simulink model "CM680A_HwTq2Meas"  (R2013b)
settings: Solver=FixedStepDiscrete  SolverMode=SingleTasking  StartTime=0.0  StopTime=1  FixedStep=0.002  RelTol=1e-3
values from neighbouring files (symbols this model uses):
  ELECGLBPRM_HWTQOFFS_HWNWTMTR_F32 = DataDict.Constant    [CM680A_HwTq2Meas_DataDict.m]
  ELECGLBPRM_HWTQSATNLOWRLIM_HWNWTMTR_F32 = DataDict.Constant    [CM680A_HwTq2Meas_DataDict.m]
  ELECGLBPRM_HWTQSATNUPPRLIM_HWNWTMTR_F32 = DataDict.Constant    [CM680A_HwTq2Meas_DataDict.m]
  ELECGLBPRM_HWTQSCA_ULS_F32 = DataDict.Constant    [CM680A_HwTq2Meas_DataDict.m]
  ELECGLBPRM_NOFLT_CNT_U08 = DataDict.Constant    [CM680A_HwTq2Meas_DataDict.m]
  ELECGLBPRM_OFFSTRIMNOTPRFM_CNT_U08 = DataDict.Constant    [CM680A_HwTq2Meas_DataDict.m]
  ELECGLBPRM_PRTCLFLT_CNT_U08 = DataDict.Constant    [CM680A_HwTq2Meas_DataDict.m]
  ELECGLBPRM_SNSRINTFLT_CNT_U08 = DataDict.Constant    [CM680A_HwTq2Meas_DataDict.m]
  FLTINJ_HWTQ2MEAS_HWTQ2 = DataDict.Constant    [CM680A_HwTq2Meas_DataDict.m]
  GearIdn1 = DataDict.OpSignal    [CM680A_HwTq2Meas_DataDict.m]
  HwTq2MeasHwTq2PrtclFltFailStep = DataDict.Calibration    [CM680A_HwTq2Meas_DataDict.m]
  HwTq2MeasHwTq2PrtclFltPassStep = DataDict.Calibration    [CM680A_HwTq2Meas_DataDict.m]
undefined symbols (not defined in the file or in its folder): NtcNr1, NtcSts1, sigbuilder_block, SigQlfr1
libraries: simulink x22, NxtrNvM x3
(part 1 of 3)
settings Model: RequirementInfo={'doors' '00006115' '1' 'false' 'DOORS Surrogate Item' '' } %GIDa_184d7b6b_0c7e_41d3_b9a0_1a88eb3981d4  reqMgrSettings="100 S'doors','misc'{{S'surrogatepath','savemodel','savesurrogate','updateLinks','doorsLinks2sl','slLinks2Doors','purgeDoors','purgeSimulink','detaillevel','surrogateId','synctime'{{T\"/ESG Group/CM660A_HwTq1Meas\",M[1],M[1],M[0],M[0],M[1],M[0],M[0],M[1],T\"00006115\",T\"\"}},S'mode','pathStorage'{{T\"generic\",T\"modelRelative\"}}}}"  CovMetricSettings=dcmriw  CovFilter=CM680A_HwTq2Meas_covfilter  CovHTMLOptions=-sRT=0 -aTS=1 -bRG=1 -bTC=1 -hTR=0 -nFC=0 -scm=1 -bcm=1 -xEv=0  CovHtmlReporting=off  CovModelRefEnable=off  Creator=CZ68DS  LastModifiedBy=CZ68DS
settings SolverCC: AutoInsertRateTranBlk=on  InsertRTBMode=Always
settings DataIOCC: LimitDataPoints=off  SaveFormat=Structure  ReturnWorkspaceOutputs=on
settings OptimizationCC: BlockReduction=off  InlineParams=on  ZeroExternalMemoryAtStartup=off  ZeroInternalMemoryAtStartup=off  OptimizeModelRefInitCode=on  LifeSpan=1
settings DebuggingCC: SignalInfNanChecking=error  SignalRangeChecking=warning  UnderspecifiedInitializationDetection=Simplified  SolverPrmCheckMsg=error  InheritedTsInSrcMsg=error  DiscreteInheritContinuousMsg=error  SingleTaskRateTransMsg=error  TasksWithSamePriorityMsg=error  SigSpecEnsureSampleTimeMsg=error  CheckMatrixSingularityMsg=error  ParameterUnderflowMsg=error  ParameterPrecisionLossMsg=error  ParameterTunabilityLossMsg=error  FixptConstUnderflowMsg=warning  FixptConstOverflowMsg=warning  VectorMatrixConversionMsg=error  SignalLabelMismatchMsg=error  UnconnectedInputMsg=error  UnconnectedOutputMsg=error  UnconnectedLineMsg=error  SFcnCompatibilityMsg=error  UniqueDataStoreMsg=warning  BusObjectLabelMismatch=error  RootOutportRequireBusObject=error  AssertControl=DisableAll  ModelReferenceIOMsg=error  ModelReferenceVersionMismatchMessage=warning  ModelReferenceIOMismatchMessage=error  ModelReferenceCSMismatchMessage=warning  ModelReferenceDataLoggingMessage=error  StateNameClashWarn=warning  StrictBusMsg=ErrorOnBusTreatedAsVector  NonBusSignalsTreatedAsBus=error  SFUnexpectedBacktrackingDiag=error  SFInvalidInputDataAccessInChartInitDiag=error  SFNoUnconditionalDefaultTransitionDiag=error  SFTransitionOutsideNaturalParentDiag=error  SFUnconditionalTransitionShadowingDiag=error  SFUndirectedBroadcastEventsDiag=error
settings ModelReferenceCC: ModelReferenceNumInstancesAllowed=Single
settings RTWCC: SystemTargetFile=autosar.tlc  GenCodeOnly=on  TemplateMakefile=ert_default_tmf  Description=AUTOSAR  GenerateReport=on  ProcessScript=autosar_make_rtw_hook  LaunchReport=on
settings CodeAppCC: GenerateComments=off  IgnoreCustomStorageClasses=off  CustomSymbolStrType=$N$R$M  CustomSymbolStrBlkIO=$N$M  SimulinkBlockComments=off
settings STFCustomTargetCC: ParMdlRefBuildCompliant=on  CompOptLevelCompliant=on  IncludeMdlTerminateFcn=off  CombineOutputUpdateFcns=on  SuppressErrorStatus=on  ERTFirstTimeCompliant=on  ERTCustomFileBanners=on  SupportNonFinite=off  SupportComplex=off  SupportContinuousTime=off  SupportNonInlinedSFcns=off  MATLABClassNameForMDSCustomization=Simulink.SoftwareTarget.ERTCustomization  AutosarCompliant=on  GRTInterface=off  SystemTargetFile=autosar.tlc
settings ERTTargetCC: CodeReplacementLibrary=ANSI_C  ConcurrentExecutionCompliant=off  IncludeMdlTerminateFcn=off  SuppressErrorStatus=on  SupportNonFinite=off  SupportComplex=off  ModelStepFunctionPrototypeControlCompliant=off  CPPClassGenCompliant=off  AutosarCompliant=on  InlinedParameterPlacement=NonHierarchical  ERTCustomFileTemplate=example_file_process.tlc  EnableUserReplacementTypes=on

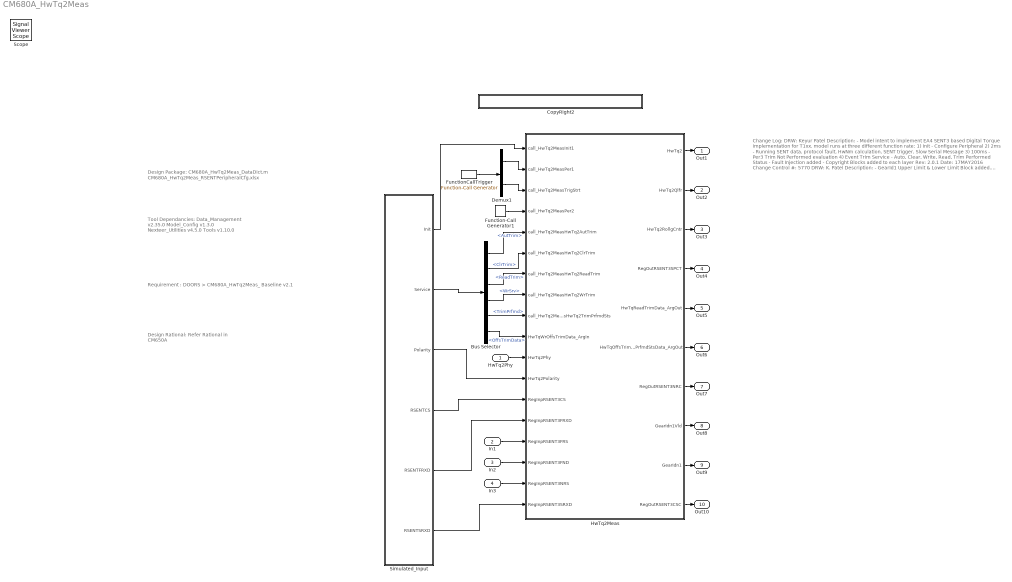
== system CM680A_HwTq2Meas ==
  note: Design Package:
      |
      | CM680A_HwTq2Meas_DataDict.m
      | CM680A_HwTq2Meas_RSENTPeripheralCfg.xlsx
  note: Change Log:
      |
      | DRW: Keyur Patel
      | Description:
      | - Model intent to implement EA4 SENT3 based Digital Torque implementation for T1xx.
      |    model runs at three different function rate:
      |       1) Init - Configure Peripheral
      |       2) 2ms - Running SENT data, protocol fault, HwNm calculation, SENT trigger, Slow Serial Message
      |       3) 100ms - Per3 Trim Not Performed evaluation
      |       4) Event Trim Service - Auto, Clear, Write, Read, Trim Performed Status
      | - Fault Injection added
      | - Copyright Blocks added to each layer
      |
      | Rev: 2.0.1
      | Date: 17MAY2016
      | Change Control #: 5770
      | DRW: K. Patel
      | Description:
      | - GearId1 Upper Limit & Lower Limit Block added.
      |
      | Rev: 2.0.0
      | Date: 15MAR2016
      | Change Control #: 4733
      | DRW: K. Patel
      | Description:
      | - Slow Serial Data Read Added for "C Factor & Bushing" signal read
      | - Timer 2us added before SPCT in NRS check added instead of SYNCM
      | - Refer Red Color High lighted Changes.
      |
      | Rev: 1.4.0
      | Date: 19JAN2016
      | Change Control #: 3376
      | DRW: K. Patel
      | Description:
      | - Refer Red Color High lighted Changes.
      | -  "CM680A_HwTq2Meas_RSENTPeripheralCfg.xlsx" change
      |
      | Rev: 1.3.0
      | Date: 16DEC2015
      | Change Control #: 3159
      | DRW: K. Patel
      | Description:
      | - Refer Red Color High lighted Changes.
      |
      | Rev: 1.2.0
      | Date: 09OCT2015
      | Change Control #: EA4#1923
      | DRW: K. Patel
      | Description:
      | - Torque Trigger server function, Per3 change to Per2, Missing Message Counter add per1,
      | remove register from "CM680A_HwTq2Meas_RSENTPeripheralCfg.xlsx", change sync time to 16
      |
      | Rev: 1.1.0
      | Date: 31JUL2015
      | Change Control #: WCR-EA4#1231
      | DRW: K. Patel
      | Description:
      | - m file correction, Tick Time change from 1us to 1.2us
      | - Global Constant
      |
      | Rev: 1.0.0
      | Date: 30JUN2015
      | Change Control #: WCR-EA4#1031
      | DRW: K. Patel
      | Description:
      | - Initial Release
      | - Fault Injection
      | - Trim Services Added
  note: Tool Dependancies:
      |
      | Data_Management v2.35.0
      | Model_Config v1.3.0
      | Nexteer_Utilities v4.5.0
      | Tools v1.10.0
  note: Requirement :
      |
      | DOORS > CM680A_HwTq2Meas_ Baseline v2.1
  note: Design Rational:
      |
      | Refer Rational in CM650A
  HwTq2Phy : Inport
  In1 : Inport  Port=2
  In2 : Inport  Port=3
  In3 : Inport  Port=4
  Bus Selector : BusSelector  OutputSignals=AutTrim,ClrTrim,ReadTrim,WrSrv,TrimPrfmd,OffsTrimData
  CopyRight2 : Subsystem  Description=|  mask(Copyright Information){none=on}
      | Copyright info block.                                               
      |                                                                     
      | Place copyright information at the top of every subsystem in design.
      mask prompts: none "No parameters"
      mask help: Place copyright information at the top of every subsystem in design.
      mask Display:
      | NxtrConf = 'Nexteer Confidential';
      | 
      | sys = bdroot; %handle for the current model ("system")
      | first = get_param(sys,'Created');
      | first = first(end-3:end);  %year is last four digits
      | 
      | last = get_param(sys,'LastModifiedDate');
      | if isempty(last)
      |     last = datestr(now,'yyyy');
      | else
      |     last = last(end-3:end);
      | end
      | 
      | if strcmp(first,last)
      |     fprintf('%s -- Copyright %s Nexteer',NxtrConf,first)
      | else
      |     fprintf('%s -- %s%s- %s Nexteer',NxtrConf,char(169),first,last)
      | end
  Demux1 : Demux  Outputs=2
  Function-Call Generator1 : simulink/Ports & Subsystems/Function-Call Generator  sample_time=0.100  numberOfIterations=1
  FunctionCallTrigger : simulink/Ports & Subsystems/Function-Call Generator  RequirementInfo={} %GIDa_461051ca_e299_4da2_91c0_e73e41056377  sample_time=0.002  numberOfIterations=1
  HwTq2Meas : Subsystem  RequirementInfo={'doors' '00006115' '2' 'false' 'DOORS Surrogate Item' '' } %GIDa_76d712c1_5f1a_450e_83af_7c4f481758f4  Priority=1
      settings: AttributesFormatString=Priority = %<Priority>
  Simulated_Input : Subsystem  Description=Do not Code this block
      settings: AttributesFormatString=%<Description>
  Out1 : Outport
  Out2 : Outport  Port=2
  Out3 : Outport  Port=3
  Out4 : Outport  Port=4
  Out5 : Outport  Port=5
  Out6 : Outport  Port=6
  Out7 : Outport  Port=7
  Out8 : Outport  Port=8
  Out9 : Outport  Port=9
  Out10 : Outport  Port=10
  Scope : SignalViewerScope  IOType=viewer  RefreshTime=0.035000
  wires:
  FunctionCallTrigger/1 -> Demux1/1
  HwTq2Phy/1 -> HwTq2Meas/11(HwTq2Phy)
  Simulated_Input/3(Polarity) -> HwTq2Meas/12(HwTq2Polarity)
  HwTq2Meas/3(HwTq2RollgCntr) -> Out3/1
  HwTq2Meas/1(HwTq2) -> Out1/1
  HwTq2Meas/2(HwTq2Qlfr) -> Out2/1
  HwTq2Meas/4(RegOutRSENT3SPCT) -> Out4/1
  Function-Call Generator1/1 -> HwTq2Meas/4(call_HwTq2MeasPer2)
  Demux1/1 -> HwTq2Meas/2(call_HwTq2MeasPer1)
  Demux1/2 -> HwTq2Meas/3(call_HwTq2MeasTrigStrt)
  Bus Selector/1 -> HwTq2Meas/5(call_HwTq2MeasHwTq2AutTrim)  "<AutTrim>"
  Bus Selector/2 -> HwTq2Meas/6(call_HwTq2MeasHwTq2ClrTrim)  "<ClrTrim>"
  Bus Selector/3 -> HwTq2Meas/7(call_HwTq2MeasHwTq2ReadTrim)  "<ReadTrim>"
  Bus Selector/4 -> HwTq2Meas/8(call_HwTq2MeasHwTq2WrTrim)  "<WrSrv>"
  Bus Selector/5 -> HwTq2Meas/9(call_HwTq2MeasHwTq2TrimPrfmdSts)  "<TrimPrfmd>"
  Bus Selector/6 -> HwTq2Meas/10(HwTqWrOffsTrimData_ArgIn)  "<OffsTrimData>"
  Simulated_Input/1(Init) -> HwTq2Meas/1(call_HwTq2MeasInit1)
  Simulated_Input/2(Service) -> Bus Selector/1
  Simulated_Input/4(RSENTCS) -> HwTq2Meas/13(RegInpRSENT3CS)
  Simulated_Input/5(RSENTFRXD) -> HwTq2Meas/14(RegInpRSENT3FRXD)
  HwTq2Meas/5(HwTqReadTrimData_ArgOut) -> Out5/1
  HwTq2Meas/6(HwTqOffsTrimPrfmdStsData_ArgOut) -> Out6/1
  HwTq2Meas/7(RegOutRSENT3NRC) -> Out7/1
  In1/1 -> HwTq2Meas/15(RegInpRSENT3FRS)
  In2/1 -> HwTq2Meas/16(RegInpRSENT3FND)
  In3/1 -> HwTq2Meas/17(RegInpRSENT3NRS)
  Simulated_Input/6(RSENTSRXD) -> HwTq2Meas/18(RegInpRSENT3SRXD)
  HwTq2Meas/8(GearIdn1Vld) -> Out8/1
  HwTq2Meas/9(GearIdn1) -> Out9/1
  HwTq2Meas/10(RegOutRSENT3CSC) -> Out10/1

== system CM680A_HwTq2Meas/CopyRight2 ==

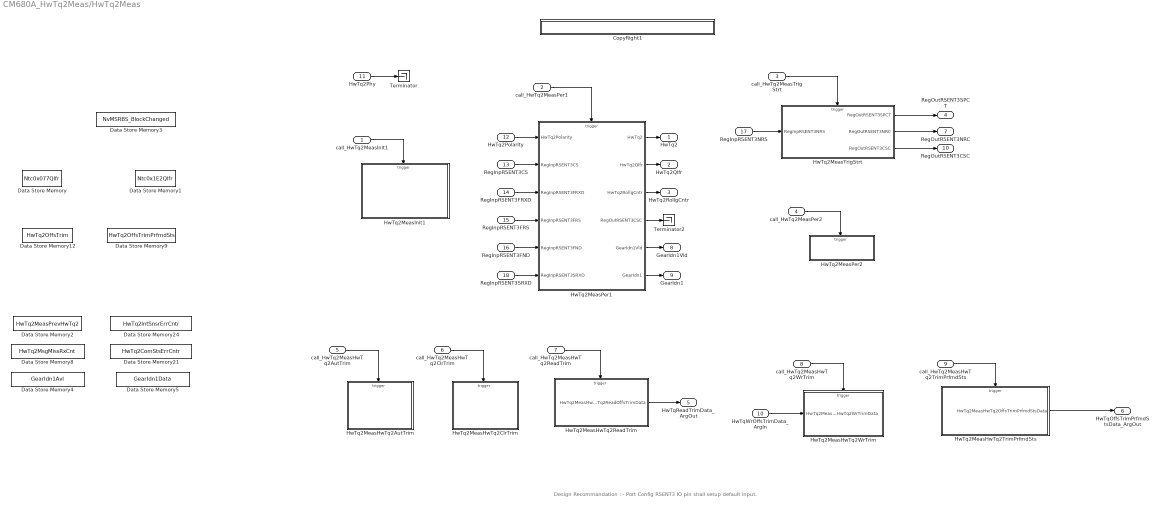
== system CM680A_HwTq2Meas/HwTq2Meas ==
  note: Design Recommandation :
      |
      | - Port Config RSENT3 IO pin shall setup default input.
  call_HwTq2MeasInit1 : Inport
  call_HwTq2MeasPer1 : Inport  Description=2ms  Port=2
      settings: AttributesFormatString=%<Description>
  call_HwTq2MeasTrigStrt : Inport  Description=Event  Port=3
      settings: AttributesFormatString=%<Description>
  call_HwTq2MeasPer2 : Inport  Description=100ms  Port=4
      settings: AttributesFormatString=%<Description>
  call_HwTq2MeasHwTq2AutTrim : Inport  Description=Event  Port=5
      settings: AttributesFormatString=%<Description>
  call_HwTq2MeasHwTq2ClrTrim : Inport  Description=Event  Port=6
      settings: AttributesFormatString=%<Description>
  call_HwTq2MeasHwTq2ReadTrim : Inport  Description=Event  Port=7
      settings: AttributesFormatString=%<Description>
  call_HwTq2MeasHwTq2WrTrim : Inport  Description=Event  Port=8
      settings: AttributesFormatString=%<Description>
  call_HwTq2MeasHwTq2TrimPrfmdSts : Inport  Description=Event  Port=9
      settings: AttributesFormatString=%<Description>
  HwTqWrOffsTrimData_ArgIn : Inport  Port=10
  HwTq2Phy : Inport  Port=11
  HwTq2Polarity : Inport  Port=12  OutDataTypeStr=int8
  RegInpRSENT3CS : Inport  Port=13
  RegInpRSENT3FRXD : Inport  Port=14
  RegInpRSENT3FRS : Inport  Port=15
  RegInpRSENT3FND : Inport  Port=16
  RegInpRSENT3NRS : Inport  Port=17
  RegInpRSENT3SRXD : Inport  Port=18
  CopyRight1 : Subsystem  Description=|  mask(Copyright Information){none=on}
      | Copyright info block.                                               
      |                                                                     
      | Place copyright information at the top of every subsystem in design.
      mask prompts: none "No parameters"
      mask help: Place copyright information at the top of every subsystem in design.
      mask Display:
      | NxtrConf = 'Nexteer Confidential';
      | 
      | sys = bdroot; %handle for the current model ("system")
      | first = get_param(sys,'Created');
      | first = first(end-3:end);  %year is last four digits
      | 
      | last = get_param(sys,'LastModifiedDate');
      | if isempty(last)
      |     last = datestr(now,'yyyy');
      | else
      |     last = last(end-3:end);
      | end
      | 
      | if strcmp(first,last)
      |     fprintf('%s -- Copyright %s Nexteer',NxtrConf,first)
      | else
      |     fprintf('%s -- %s%s- %s Nexteer',NxtrConf,char(169),first,last)
      | end
  Data Store Memory12 : DataStoreMemory  DataStoreName=HwTq2OffsTrim  ReadBeforeWriteMsg=warning  WriteAfterWriteMsg=warning  WriteAfterReadMsg=warning
  Data Store Memory2 : DataStoreMemory  DataStoreName=HwTq2MeasPrevHwTq2  ReadBeforeWriteMsg=warning  WriteAfterWriteMsg=warning  WriteAfterReadMsg=warning  StateMustResolveToSignalObject=on
  Data Store Memory21 : DataStoreMemory  DataStoreName=HwTq2ComStsErrCntr  ReadBeforeWriteMsg=warning  WriteAfterWriteMsg=warning  WriteAfterReadMsg=warning  StateMustResolveToSignalObject=on
  Data Store Memory24 : DataStoreMemory  DataStoreName=HwTq2IntSnsrErrCntr  ReadBeforeWriteMsg=warning  WriteAfterWriteMsg=warning  WriteAfterReadMsg=warning  StateMustResolveToSignalObject=on
  Data Store Memory4 : DataStoreMemory  DataStoreName=GearIdn1Avl  ReadBeforeWriteMsg=warning  WriteAfterWriteMsg=warning  WriteAfterReadMsg=warning  StateMustResolveToSignalObject=on
  Data Store Memory5 : DataStoreMemory  DataStoreName=GearIdn1Data  ReadBeforeWriteMsg=warning  WriteAfterWriteMsg=warning  WriteAfterReadMsg=warning  StateMustResolveToSignalObject=on
  Data Store Memory8 : DataStoreMemory  DataStoreName=HwTq2MsgMissRxCnt  ReadBeforeWriteMsg=warning  WriteAfterWriteMsg=warning  WriteAfterReadMsg=warning  StateMustResolveToSignalObject=on
  Data Store Memory9 : DataStoreMemory  DataStoreName=HwTq2OffsTrimPrfmdSts  ReadBeforeWriteMsg=warning  WriteAfterWriteMsg=warning  WriteAfterReadMsg=warning
  Data Store Memory : DataStoreMemory  DataStoreName=Ntc0x077Qlfr  ReadBeforeWriteMsg=warning  WriteAfterWriteMsg=warning  WriteAfterReadMsg=warning  OutDataTypeStr=uint8
      settings: AttributesFormatString=|
      | Simulation Purpose Only.
      | Do Not Code this block
      | Diagnostic Manager Owns this requirement
  Data Store Memory1 : DataStoreMemory  DataStoreName=Ntc0x1E2Qlfr  ReadBeforeWriteMsg=warning  WriteAfterWriteMsg=warning  WriteAfterReadMsg=warning  OutDataTypeStr=uint8
      settings: AttributesFormatString=|
      | Simulation Purpose Only.
      | Do Not Code this block
      | Diagnostic Manager Owns this requirement
  Data Store Memory3 : DataStoreMemory  DataStoreName=NvMSRBS_BlockChanged  ReadBeforeWriteMsg=warning  WriteAfterWriteMsg=warning  WriteAfterReadMsg=warning  OutDataTypeStr=uint8
      settings: AttributesFormatString=|
      | Simulation Purpose Only.
      | Do Not Code this block
      | Diagnostic Manager Owns this requirement
  HwTq2MeasHwTq2AutTrim : Subsystem  RequirementInfo={'linktype_rmi_doors' '0000cf42 (/ESG Group/FDD Module Requirements/EA4 Specific/CM680A_HwTq2Meas)' '#CM680A_57' 'true' 'REQ: CM680A_57' '' } %GIDa_78a0150d_b2b2_4893_8cf0_7a267cd87682  Priority=10  TreatAsAtomicUnit=on
      settings: AttributesFormatString=Priority=%<Priority>
  HwTq2MeasHwTq2ClrTrim : Subsystem  RequirementInfo={'linktype_rmi_doors' '0000cf42 (/ESG Group/FDD Module Requirements/EA4 Specific/CM680A_HwTq2Meas)' '#CM680A_55' 'true' 'REQ: CM680A_55' '' } %GIDa_9d8bf3ad_e540_4a5e_ad4c_eb940ac157ad  Priority=10  TreatAsAtomicUnit=on
      settings: AttributesFormatString=Priority=%<Priority>
  HwTq2MeasHwTq2ReadTrim : Subsystem  RequirementInfo={'linktype_rmi_doors' '0000cf42 (/ESG Group/FDD Module Requirements/EA4 Specific/CM680A_HwTq2Meas)' '#CM680A_53' 'true' 'REQ: CM680A_53' '' } %GIDa_4c78535b_9e38_436f_a670_46438fd62cfe  Priority=10  TreatAsAtomicUnit=on
      settings: AttributesFormatString=Priority=%<Priority>
  HwTq2MeasHwTq2TrimPrfmdSts : Subsystem  RequirementInfo={'linktype_rmi_doors' '0000cf42 (/ESG Group/FDD Module Requirements/EA4 Specific/CM680A_HwTq2Meas)' '#CM680A_54' 'true' 'REQ: CM680A_54' '' } %GIDa_05e70ef2_f8d5_471c_a4a3_b95d94c92180  Priority=10  TreatAsAtomicUnit=on
      settings: AttributesFormatString=Priority=%<Priority>
  HwTq2MeasHwTq2WrTrim : Subsystem  RequirementInfo={'linktype_rmi_doors' '0000cf42 (/ESG Group/FDD Module Requirements/EA4 Specific/CM680A_HwTq2Meas)' '#CM680A_56' 'true' 'REQ: CM680A_56' '' } %GIDa_58f23a20_9e17_4252_b727_77362ca5c7be  Priority=10  TreatAsAtomicUnit=on
      settings: AttributesFormatString=Priority=%<Priority>
  HwTq2MeasInit1 : Subsystem  TreatAsAtomicUnit=on
  HwTq2MeasPer1 : Subsystem  RequirementInfo={'linktype_rmi_doors' '0000cf42 (/ESG Group/FDD Module Requirements/EA4 Specific/CM680A_HwTq2Meas)' '#CM680A_27' 'true' 'REQ: CM680A_27' '' ; 'linktype_rmi_doors' '0000cf42 (/ESG Group/FDD Module Requirements/EA4 Specific/CM680A_HwTq2Meas)' '#CM680A_39' 'true' 'REQ: CM680A_39' '' } %GIDa_31b3da74_5937_4fb2_b915_5c5c5e5711e7  TreatAsAtomicUnit=on
  HwTq2MeasPer2 : Subsystem  RequirementInfo={'linktype_rmi_doors' '0000cf42 (/ESG Group/FDD Module Requirements/EA4 Specific/CM680A_HwTq2Meas)' '#CM680A_62' 'true' 'REQ: CM680A_62' '' } %GIDa_c89b04b6_b4c1_41bf_b3f8_efad30b9fb82  Priority=8  TreatAsAtomicUnit=on
      settings: AttributesFormatString=Priority=%<Priority>
  HwTq2MeasTrigStrt : Subsystem  RequirementInfo={'linktype_rmi_doors' '0000cf42 (/ESG Group/FDD Module Requirements/EA4 Specific/CM680A_HwTq2Meas)' '#CM680A_33' 'true' 'REQ: CM680A_33' '' } %GIDa_ac2e4248_233e_47e7_8dc6_e55969fb5c4e  TreatAsAtomicUnit=on
  Terminator : Terminator
  Terminator2 : Terminator
  HwTq2 : Outport
  HwTq2Qlfr : Outport  Port=2
  HwTq2RollgCntr : Outport  Port=3
  RegOutRSENT3SPCT : Outport  Port=4
  HwTqReadTrimData_ArgOut : Outport  Port=5
  HwTqOffsTrimPrfmdStsData_ArgOut : Outport  Port=6
  RegOutRSENT3NRC : Outport  Port=7
  GearIdn1Vld : Outport  Port=8
  GearIdn1 : Outport  Port=9
  RegOutRSENT3CSC : Outport  Port=10
  wires:
  call_HwTq2MeasPer1/1 -> HwTq2MeasPer1/Trigger
  call_HwTq2MeasInit1/1 -> HwTq2MeasInit1/Trigger
  HwTq2MeasPer1/1(HwTq2) -> HwTq2/1
  HwTq2MeasPer1/2(HwTq2Qlfr) -> HwTq2Qlfr/1
  HwTq2MeasPer1/3(HwTq2RollgCntr) -> HwTq2RollgCntr/1
  call_HwTq2MeasTrigStrt/1 -> HwTq2MeasTrigStrt/Trigger
  HwTq2Polarity/1 -> HwTq2MeasPer1/1(HwTq2Polarity)
  HwTq2MeasTrigStrt/1(RegOutRSENT3SPCT) -> RegOutRSENT3SPCT/1
  HwTq2Phy/1 -> Terminator/1
  call_HwTq2MeasHwTq2AutTrim/1 -> HwTq2MeasHwTq2AutTrim/Trigger
  call_HwTq2MeasHwTq2ClrTrim/1 -> HwTq2MeasHwTq2ClrTrim/Trigger
  call_HwTq2MeasHwTq2ReadTrim/1 -> HwTq2MeasHwTq2ReadTrim/Trigger
  call_HwTq2MeasHwTq2WrTrim/1 -> HwTq2MeasHwTq2WrTrim/Trigger
  call_HwTq2MeasHwTq2TrimPrfmdSts/1 -> HwTq2MeasHwTq2TrimPrfmdSts/Trigger
  HwTqWrOffsTrimData_ArgIn/1 -> HwTq2MeasHwTq2WrTrim/1(HwTq2MeasHwTq2WrTrimData)
  HwTq2MeasHwTq2ReadTrim/1(HwTq2MeasHwTq2ReadOffsTrimData) -> HwTqReadTrimData_ArgOut/1
  HwTq2MeasHwTq2TrimPrfmdSts/1(HwTq2MeasHwTq2OffsTrimPrfmdStsData) -> HwTqOffsTrimPrfmdStsData_ArgOut/1
  call_HwTq2MeasPer2/1 -> HwTq2MeasPer2/Trigger
  RegInpRSENT3CS/1 -> HwTq2MeasPer1/2(RegInpRSENT3CS)
  RegInpRSENT3FND/1 -> HwTq2MeasPer1/5(RegInpRSENT3FND)
  RegInpRSENT3FRS/1 -> HwTq2MeasPer1/4(RegInpRSENT3FRS)
  RegInpRSENT3FRXD/1 -> HwTq2MeasPer1/3(RegInpRSENT3FRXD)
  HwTq2MeasPer1/4(RegOutRSENT3CSC) -> Terminator2/1
  RegInpRSENT3NRS/1 -> HwTq2MeasTrigStrt/1(RegInpRSENT3NRS)
  HwTq2MeasTrigStrt/3(RegOutRSENT3CSC) -> RegOutRSENT3CSC/1
  HwTq2MeasTrigStrt/2(RegOutRSENT3NRC) -> RegOutRSENT3NRC/1
  RegInpRSENT3SRXD/1 -> HwTq2MeasPer1/6(RegInpRSENT3SRXD)
  HwTq2MeasPer1/6(GearIdn1) -> GearIdn1/1
  HwTq2MeasPer1/5(GearIdn1Vld) -> GearIdn1Vld/1

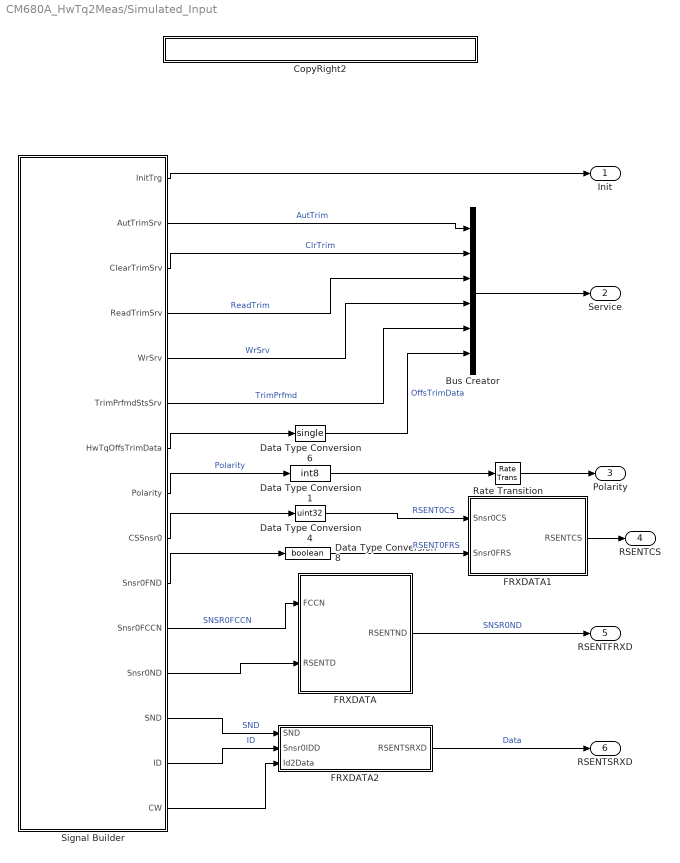
== system CM680A_HwTq2Meas/Simulated_Input ==
  Bus Creator : BusCreator  Inputs=6
  CopyRight2 : Subsystem  Description=|  mask(Copyright Information){none=on}
      | Copyright info block.                                               
      |                                                                     
      | Place copyright information at the top of every subsystem in design.
      mask prompts: none "No parameters"
      mask help: Place copyright information at the top of every subsystem in design.
      mask Display:
      | NxtrConf = 'Nexteer Confidential';
      | 
      | sys = bdroot; %handle for the current model ("system")
      | first = get_param(sys,'Created');
      | first = first(end-3:end);  %year is last four digits
      | 
      | last = get_param(sys,'LastModifiedDate');
      | if isempty(last)
      |     last = datestr(now,'yyyy');
      | else
      |     last = last(end-3:end);
      | end
      | 
      | if strcmp(first,last)
      |     fprintf('%s -- Copyright %s Nexteer',NxtrConf,first)
      | else
      |     fprintf('%s -- %s%s- %s Nexteer',NxtrConf,char(169),first,last)
      | end
  Data Type Conversion1 : DataTypeConversion  OutDataTypeStr=int8
  Data Type Conversion4 : DataTypeConversion  OutDataTypeStr=uint32
  Data Type Conversion6 : DataTypeConversion  OutDataTypeStr=single
  Data Type Conversion8 : DataTypeConversion  OutDataTypeStr=boolean
  FRXDATA : Subsystem
  FRXDATA1 : Subsystem
  FRXDATA2 : Subsystem
  Rate Transition : RateTransition
  Signal Builder : Subsystem  Tag=STV Subsys  LoadFcn=sigbuilder_block('load');  StartFcn=sigbuilder_block('start');  StopFcn=sigbuilder_block('stop');  ClipboardFcn=sigbuilder_block('clipboard');  mask(Sigbuilder block){}
      mask help: Simulink:masks:SigbuilderBlock_MD
      mask init:
      | if ~strcmp(get_param(bdroot(gcbh),'SimulationStatus'),'stopped') tuvar = sigbuilder_block('maskInit'); end
      settings: CopyFcn=sigbuilder_block('copy');  DeleteFcn=sigbuilder_block('delete');  ModelCloseFcn=sigbuilder_block('modelClose');  PreSaveFcn=sigbuilder_block('preSave');  PauseFcn=sigbuilder_block('pause');  ContinueFcn=sigbuilder_block('continue');  NameChangeFcn=sigbuilder_block('namechange');  OpenFcn=sigbuilder_block('open',[339.75 708 961.5 507 ]);  CloseFcn=sigbuilder_block('close');
      mask Display: plot(0, 0, 100, 100,[2, 2, 32, 32, 2], [68, 8, 8, 68, 68],[32, 2], [38, 38], [32, 19, 2],[53, 60, 44], [32, 17, 17, 2],[16, 16, 31, 31]);txt = getActiveGroup(gcbh);text(2, 100, txt,'verticalAlignment', 'top');
  Init : Outport
  Service : Outport  Port=2
  Polarity : Outport  Port=3
  RSENTCS : Outport  Port=4
  RSENTFRXD : Outport  Port=5
  RSENTSRXD : Outport  Port=6
  wires:
  FRXDATA1/1(RSENTCS) -> RSENTCS/1
  Signal Builder/15(CW) -> FRXDATA2/3(Id2Data)
  Signal Builder/14(ID) -> FRXDATA2/2(Snsr0IDD)  "ID"
  FRXDATA2/1(RSENTSRXD) -> RSENTSRXD/1  "Data"
  Signal Builder/13(SND) -> FRXDATA2/1(SND)  "SND"
  Signal Builder/8(Polarity) -> Data Type Conversion1/1  "Polarity"
  Signal Builder/1(InitTrg) -> Init/1
  Signal Builder/7(HwTqOffsTrimData) -> Data Type Conversion6/1
  Signal Builder/6(TrimPrfmdStsSrv) -> Bus Creator/5  "TrimPrfmd"
  Signal Builder/5(WrSrv) -> Bus Creator/4  "WrSrv"
  Signal Builder/4(ReadTrimSrv) -> Bus Creator/3  "ReadTrim"
  Signal Builder/3(ClearTrimSrv) -> Bus Creator/2  "ClrTrim"
  Signal Builder/2(AutTrimSrv) -> Bus Creator/1  "AutTrim"
  Signal Builder/12(Snsr0ND) -> FRXDATA/2(RSENTD)
  Signal Builder/9(CSSnsr0) -> Data Type Conversion4/1
  Signal Builder/10(Snsr0FND) -> Data Type Conversion8/1
  Bus Creator/1 -> Service/1
  FRXDATA/1(RSENTND) -> RSENTFRXD/1  "SNSR0ND"
  Data Type Conversion1/1 -> Rate Transition/1
  Rate Transition/1 -> Polarity/1
  Data Type Conversion4/1 -> FRXDATA1/1(Snsr0CS)  "RSENT0CS"
  Data Type Conversion8/1 -> FRXDATA1/2(Snsr0FRS)  "RSENT0FRS"
  Signal Builder/11(Snsr0FCCN) -> FRXDATA/1(FCCN)  "SNSR0FCCN"
  Data Type Conversion6/1 -> Bus Creator/6  "OffsTrimData"

== system CM680A_HwTq2Meas/HwTq2Meas/CopyRight1 ==

== system CM680A_HwTq2Meas/HwTq2Meas/HwTq2MeasHwTq2AutTrim ==
  function : TriggerPort
  CopyRight2 : Subsystem  Description=|  mask(Copyright Information){none=on}
      | Copyright info block.                                               
      |                                                                     
      | Place copyright information at the top of every subsystem in design.
      mask prompts: none "No parameters"
      mask help: Place copyright information at the top of every subsystem in design.
      mask Display:
      | NxtrConf = 'Nexteer Confidential';
      | 
      | sys = bdroot; %handle for the current model ("system")
      | first = get_param(sys,'Created');
      | first = first(end-3:end);  %year is last four digits
      | 
      | last = get_param(sys,'LastModifiedDate');
      | if isempty(last)
      |     last = datestr(now,'yyyy');
      | else
      |     last = last(end-3:end);
      | end
      | 
      | if strcmp(first,last)
      |     fprintf('%s -- Copyright %s Nexteer',NxtrConf,first)
      | else
      |     fprintf('%s -- %s%s- %s Nexteer',NxtrConf,char(169),first,last)
      | end
  NVM Shadow RAM : DataStoreWrite  RequirementInfo={} %GIDa_691c2588_2b45_48b9_9733_fd18f25444bb  DataStoreName=HwTq2OffsTrim
  NVM1 Shadow RAM : DataStoreWrite  RequirementInfo={'linktype_rmi_doors' '0000cf42 (/ESG Group/FDD Module Requirements/EA4 Specific/CM680A_HwTq2Meas)' '#CM680A_50' 'true' 'REQ: CM680A_50' '' } %GIDa_8dfe2b68_c9bd_4b5f_9a85_4945a725dea6  DataStoreName=HwTq2OffsTrimPrfmdSts
  PIM : DataStoreRead  RequirementInfo={} %GIDa_7720d852_cab6_4ee8_822b_ee5ddb596286  Priority=10  DataStoreName=HwTq2MeasPrevHwTq2
      settings: AttributesFormatString=Priority=%<Priority>
  Set : Constant
  Set Ram Block Status : NxtrNvM/Set Ram Block Status  FuncName=Set Ram Block Status  NvMBlockName=HwTq2Offs  VoidFuncRtn=on  BlockChanged_DSN=NvMSRBS_BlockChanged  Return_DSN=NvMSRBS_Return
      settings: AttributesFormatString=%<FuncName>
  Set3 : Constant  OutDataTypeStr=uint8
  wires:
  PIM/1 -> NVM Shadow RAM/1
  Set/1 -> NVM1 Shadow RAM/1
  Set3/1 -> Set Ram Block Status/1

== system CM680A_HwTq2Meas/HwTq2Meas/HwTq2MeasHwTq2ClrTrim ==
  function : TriggerPort
  Clear1 : Constant  Value=0  OutDataTypeStr=single
  Clear2 : Constant  Value=0
  CopyRight2 : Subsystem  Description=|  mask(Copyright Information){none=on}
      | Copyright info block.                                               
      |                                                                     
      | Place copyright information at the top of every subsystem in design.
      mask prompts: none "No parameters"
      mask help: Place copyright information at the top of every subsystem in design.
      mask Display:
      | NxtrConf = 'Nexteer Confidential';
      | 
      | sys = bdroot; %handle for the current model ("system")
      | first = get_param(sys,'Created');
      | first = first(end-3:end);  %year is last four digits
      | 
      | last = get_param(sys,'LastModifiedDate');
      | if isempty(last)
      |     last = datestr(now,'yyyy');
      | else
      |     last = last(end-3:end);
      | end
      | 
      | if strcmp(first,last)
      |     fprintf('%s -- Copyright %s Nexteer',NxtrConf,first)
      | else
      |     fprintf('%s -- %s%s- %s Nexteer',NxtrConf,char(169),first,last)
      | end
  NVM Shadow RAM : DataStoreWrite  RequirementInfo={} %GIDa_c01938bd_873a_4f20_8aad_b7368db2e426  DataStoreName=HwTq2OffsTrim
  NVM1 Shadow RAM : DataStoreWrite  RequirementInfo={'linktype_rmi_doors' '0000cf42 (/ESG Group/FDD Module Requirements/EA4 Specific/CM680A_HwTq2Meas)' '#CM680A_50' 'true' 'REQ: CM680A_50' '' } %GIDa_7e661117_be14_43c5_b4c7_51bd14c3b186  DataStoreName=HwTq2OffsTrimPrfmdSts
  Set Ram Block Status : NxtrNvM/Set Ram Block Status  FuncName=Set Ram Block Status  NvMBlockName=HwTq2Offs  VoidFuncRtn=on  BlockChanged_DSN=NvMSRBS_BlockChanged  Return_DSN=NvMSRBS_Return
      settings: AttributesFormatString=%<FuncName>
  Set3 : Constant  OutDataTypeStr=uint8
  wires:
  Clear1/1 -> NVM Shadow RAM/1
  Clear2/1 -> NVM1 Shadow RAM/1
  Set3/1 -> Set Ram Block Status/1

== system CM680A_HwTq2Meas/HwTq2Meas/HwTq2MeasHwTq2ReadTrim ==
  function : TriggerPort
  CopyRight2 : Subsystem  Description=|  mask(Copyright Information){none=on}
      | Copyright info block.                                               
      |                                                                     
      | Place copyright information at the top of every subsystem in design.
      mask prompts: none "No parameters"
      mask help: Place copyright information at the top of every subsystem in design.
      mask Display:
      | NxtrConf = 'Nexteer Confidential';
      | 
      | sys = bdroot; %handle for the current model ("system")
      | first = get_param(sys,'Created');
      | first = first(end-3:end);  %year is last four digits
      | 
      | last = get_param(sys,'LastModifiedDate');
      | if isempty(last)
      |     last = datestr(now,'yyyy');
      | else
      |     last = last(end-3:end);
      | end
      | 
      | if strcmp(first,last)
      |     fprintf('%s -- Copyright %s Nexteer',NxtrConf,first)
      | else
      |     fprintf('%s -- %s%s- %s Nexteer',NxtrConf,char(169),first,last)
      | end
  NVM Shadow RAM : DataStoreRead  DataStoreName=HwTq2OffsTrim
  HwTq2MeasHwTq2ReadOffsTrimData : Outport
  wires:
  NVM Shadow RAM/1 -> HwTq2MeasHwTq2ReadOffsTrimData/1

== system CM680A_HwTq2Meas/HwTq2Meas/HwTq2MeasHwTq2TrimPrfmdSts ==
  function : TriggerPort
  CopyRight2 : Subsystem  Description=|  mask(Copyright Information){none=on}
      | Copyright info block.                                               
      |                                                                     
      | Place copyright information at the top of every subsystem in design.
      mask prompts: none "No parameters"
      mask help: Place copyright information at the top of every subsystem in design.
      mask Display:
      | NxtrConf = 'Nexteer Confidential';
      | 
      | sys = bdroot; %handle for the current model ("system")
      | first = get_param(sys,'Created');
      | first = first(end-3:end);  %year is last four digits
      | 
      | last = get_param(sys,'LastModifiedDate');
      | if isempty(last)
      |     last = datestr(now,'yyyy');
      | else
      |     last = last(end-3:end);
      | end
      | 
      | if strcmp(first,last)
      |     fprintf('%s -- Copyright %s Nexteer',NxtrConf,first)
      | else
      |     fprintf('%s -- %s%s- %s Nexteer',NxtrConf,char(169),first,last)
      | end
  Data Store Read1 : DataStoreRead  DataStoreName=HwTq2OffsTrimPrfmdSts
  HwTq2MeasHwTq2OffsTrimPrfmdStsData : Outport
  wires:
  Data Store Read1/1 -> HwTq2MeasHwTq2OffsTrimPrfmdStsData/1

== system CM680A_HwTq2Meas/HwTq2Meas/HwTq2MeasHwTq2WrTrim ==
  HwTq2MeasHwTq2WrTrimData : Inport
  function : TriggerPort
  CopyRight2 : Subsystem  Description=|  mask(Copyright Information){none=on}
      | Copyright info block.                                               
      |                                                                     
      | Place copyright information at the top of every subsystem in design.
      mask prompts: none "No parameters"
      mask help: Place copyright information at the top of every subsystem in design.
      mask Display:
      | NxtrConf = 'Nexteer Confidential';
      | 
      | sys = bdroot; %handle for the current model ("system")
      | first = get_param(sys,'Created');
      | first = first(end-3:end);  %year is last four digits
      | 
      | last = get_param(sys,'LastModifiedDate');
      | if isempty(last)
      |     last = datestr(now,'yyyy');
      | else
      |     last = last(end-3:end);
      | end
      | 
      | if strcmp(first,last)
      |     fprintf('%s -- Copyright %s Nexteer',NxtrConf,first)
      | else
      |     fprintf('%s -- %s%s- %s Nexteer',NxtrConf,char(169),first,last)
      | end
  NVM Shadow RAM : DataStoreWrite  RequirementInfo={} %GIDa_1659f01a_6b97_4ff1_afb0_e4ba99927e44  DataStoreName=HwTq2OffsTrim
  NVM1 Shadow RAM : DataStoreWrite  RequirementInfo={'linktype_rmi_doors' '0000cf42 (/ESG Group/FDD Module Requirements/EA4 Specific/CM680A_HwTq2Meas)' '#CM680A_50' 'true' 'REQ: CM680A_50' '' } %GIDa_340e34c7_c59a_43cb_a8d9_5aafb58ec96b  DataStoreName=HwTq2OffsTrimPrfmdSts
  Set : Constant
  Set Ram Block Status : NxtrNvM/Set Ram Block Status  FuncName=Set Ram Block Status  NvMBlockName=HwTq2Offs  VoidFuncRtn=on  BlockChanged_DSN=NvMSRBS_BlockChanged  Return_DSN=NvMSRBS_Return
      settings: AttributesFormatString=%<FuncName>
  Set3 : Constant  OutDataTypeStr=uint8
  wires:
  Set/1 -> NVM1 Shadow RAM/1
  HwTq2MeasHwTq2WrTrimData/1 -> NVM Shadow RAM/1
  Set3/1 -> Set Ram Block Status/1

== system CM680A_HwTq2Meas/HwTq2Meas/HwTq2MeasInit1 ==
  note: Follow below steps in same order:
      |
      | 1. Enable Configuration mode, RSENT3MDC.OMC = 1U
      | 2. Verify whether peripheral is in Configuration mode RSENT3MST.OMS ==1U and wait till 2us* ,it is in configuration mode
      | 3. Configure the SENT Register as per  "CM680A_HwTq2Meas_RSENTPeripheralCfg.xlsx"
      | 4. Enable Operation active mode, RSENT3MDC.OMC = 5U
      | 5. Verify whether peripheral is in Opertation active mode RSENT3MST.OMS ==5U and wait till 2us* ,it is in Opertation active mode
      | 6. Client Call "IoHwAb_SetFctPrphlHwTq2"- Port Configuration shall change to output in alternate mode from default input for RSENT3 SPCO IO pin.
      |
      | Note: * - actual minimum is 150ns as per Scott Winder email from Renesas
  function : TriggerPort  TriggerType=falling
  CopyRight2 : Subsystem  Description=|  mask(Copyright Information){none=on}
      | Copyright info block.                                               
      |                                                                     
      | Place copyright information at the top of every subsystem in design.
      mask prompts: none "No parameters"
      mask help: Place copyright information at the top of every subsystem in design.
      mask Display:
      | NxtrConf = 'Nexteer Confidential';
      | 
      | sys = bdroot; %handle for the current model ("system")
      | first = get_param(sys,'Created');
      | first = first(end-3:end);  %year is last four digits
      | 
      | last = get_param(sys,'LastModifiedDate');
      | if isempty(last)
      |     last = datestr(now,'yyyy');
      | else
      |     last = last(end-3:end);
      | end
      | 
      | if strcmp(first,last)
      |     fprintf('%s -- Copyright %s Nexteer',NxtrConf,first)
      | else
      |     fprintf('%s -- %s%s- %s Nexteer',NxtrConf,char(169),first,last)
      | end
  GetRefTmr1MicroSec32bit : Subsystem
      settings: AttributesFormatString=Client Call : Start Time
  GetTiSpan1MicroSec32bit : Subsystem
  IoHwAb_SetFctPrphlHwTq2 : Subsystem
  Terminator1 : Terminator
  wires:
  GetRefTmr1MicroSec32bit/1(RefTmr) -> GetTiSpan1MicroSec32bit/1(RefTmr)
  GetTiSpan1MicroSec32bit/1(TiSpan) -> Terminator1/1

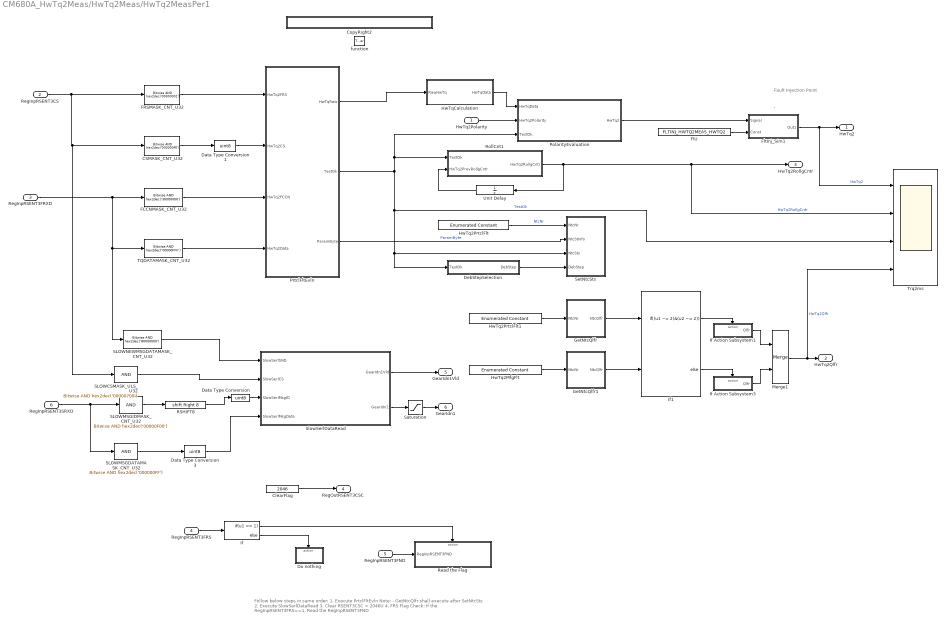
== system CM680A_HwTq2Meas/HwTq2Meas/HwTq2MeasPer1 ==
  note: ,
  note: Fault
      | Injection
      | Point
  note: Follow below steps in same order:
      |
      | 1. Execute PrtclFltEvln
      | Note: - GetNtcQlfr shall execute after SetNtcSts
      | 2. Execute SlowSerlDataRead
      |
      | 3. Clear RSENT3CSC = 2046U
      | 4. FRS Flag Check: If the RegInpRSENT3FRS==1,  Read the RegInpRSENT3FND
  HwTq2Polarity : Inport
  RegInpRSENT3CS : Inport  Port=2
  RegInpRSENT3FRXD : Inport  Port=3
  RegInpRSENT3FRS : Inport  Port=4
  RegInpRSENT3FND : Inport  Port=5
  RegInpRSENT3SRXD : Inport  Port=6
  function : TriggerPort  TriggerType=function-call
  CSMASK_CNT_U32 : simulink/Logic and Bit Operations/Bitwise Operator  logicop=AND  UseBitMask=on  BitMask=hex2dec('000000FE')  BitMaskRealWorld=Stored Integer
  ClearFlag : Constant  RequirementInfo={} %GIDa_818d7055_d423_4342_aa49_e4e3b3395427  Value=2046  OutDataTypeStr=uint16
  CopyRight2 : Subsystem  Description=|  mask(Copyright Information){none=on}
      | Copyright info block.                                               
      |                                                                     
      | Place copyright information at the top of every subsystem in design.
      mask prompts: none "No parameters"
      mask help: Place copyright information at the top of every subsystem in design.
      mask Display:
      | NxtrConf = 'Nexteer Confidential';
      | 
      | sys = bdroot; %handle for the current model ("system")
      | first = get_param(sys,'Created');
      | first = first(end-3:end);  %year is last four digits
      | 
      | last = get_param(sys,'LastModifiedDate');
      | if isempty(last)
      |     last = datestr(now,'yyyy');
      | else
      |     last = last(end-3:end);
      | end
      | 
      | if strcmp(first,last)
      |     fprintf('%s -- Copyright %s Nexteer',NxtrConf,first)
      | else
      |     fprintf('%s -- %s%s- %s Nexteer',NxtrConf,char(169),first,last)
      | end
  Data Type Conversion : DataTypeConversion  OutDataTypeStr=uint8
  Data Type Conversion1 : DataTypeConversion  OutDataTypeStr=uint8
  Data Type Conversion3 : DataTypeConversion  OutDataTypeStr=uint8
  DebStepSelection : Subsystem
  Do nothing : Subsystem  RequirementInfo={} %GIDa_95c55341_7751_4892_9e2a_824303ad0793  TreatAsAtomicUnit=on
  FCCNMASK_CNT_U32 : simulink/Logic and Bit Operations/Bitwise Operator  logicop=AND  UseBitMask=on  BitMask=hex2dec('30000000')  BitMaskRealWorld=Stored Integer
  FIU : Constant  Value=FLTINJ_HWTQ2MEAS_HWTQ2
  FRSMASK_CNT_U32 : simulink/Logic and Bit Operations/Bitwise Operator  logicop=AND  UseBitMask=on  BitMask=hex2dec('00000001')  BitMaskRealWorld=Stored Integer
  FltInj_Sim1 : Subsystem  RequirementInfo={'linktype_rmi_doors' '0000cf42 (/ESG Group/FDD Module Requirements/EA4 Specific/CM680A_HwTq2Meas)' '#CM680A_51' 'true' 'REQ: CM680A_51' '' } %GIDa_134aebb3_cf60_4723_aef6_c3de81ab27af  TreatAsAtomicUnit=on  VariantControl=FltInj_sim  mask(Fault_Injection){}
      mask help: Fault Injection is a simulation only block for EA4 programs.
  GetNtcQlfr : Subsystem
  GetNtcQlfr1 : Subsystem
  HwTq2MfgFlt : simulink/Sources/Enumerated Constant  OutDataTypeStr=Enum: NtcNr1  Value=NtcNr1.NTCNR_0X1E2  SampleTime=inf
  HwTq2PrtclFlt : simulink/Sources/Enumerated Constant  OutDataTypeStr=Enum: NtcNr1  Value=NtcNr1.NTCNR_0X077  SampleTime=inf
  HwTq2PrtclFlt1 : simulink/Sources/Enumerated Constant  OutDataTypeStr=Enum: NtcNr1  Value=NtcNr1.NTCNR_0X077  SampleTime=inf
  HwTqCalculation : Subsystem
  If : If  RequirementInfo={} %GIDa_bfa578f4_d892_42dc_8f30_1348bbb553d3  IfExpression=u1 == 1
  If Action Subsystem1 : Subsystem  TreatAsAtomicUnit=on
  If Action Subsystem3 : Subsystem  TreatAsAtomicUnit=on
  If1 : If  NumInputs=2  IfExpression=(u1 ~= 2)&(u2 ~= 2)
  Merge1 : Merge
  PolarityEvaluation : Subsystem  RequirementInfo={'linktype_rmi_doors' '0000cf42 (/ESG Group/FDD Module Requirements/EA4 Specific/CM680A_HwTq2Meas)' '#CM680A_29' 'true' 'REQ: CM680A_29' '' ; 'linktype_rmi_doors' '0000cf42 (/ESG Group/FDD Module Requirements/EA4 Specific/CM680A_HwTq2Meas)' '#CM680A_32' 'true' 'REQ: CM680A_32' '' } %GIDa_7dd0f124_da9d_41af_bfd5_c8f0b8205e28
  PrtclFltEvln : Subsystem  RequirementInfo={'doors' '00006115' '16' 'false' 'DOORS Surrogate Item' '' } %GIDa_9ddede9b_2ee1_447b_ab8b_835557d5d4fb
  RSHIFT8 : ArithShift  BitShiftNumber=8  BitShiftDirection=Right
  Read the Flag : Subsystem  RequirementInfo={} %GIDa_5c074145_5040_484b_844e_ef3bb0582b10  TreatAsAtomicUnit=on
  RollCnt1 : Stateflow chart  RequirementInfo={} %GIDa_be1c412e_1791_4e7e_9b3e_cc09ba9a6629  TreatAsAtomicUnit=on
  SLOWCSMASK_ULS_U32 : simulink/Logic and Bit Operations/Bitwise Operator  logicop=AND  UseBitMask=on  BitMask=hex2dec('00000700')  BitMaskRealWorld=Stored Integer
  SLOWMSGDATAMASK_CNT_U32 : simulink/Logic and Bit Operations/Bitwise Operator  logicop=AND  UseBitMask=on  BitMask=hex2dec('000000FF')  BitMaskRealWorld=Stored Integer
  SLOWMSGIDMASK_CNT_U32 : simulink/Logic and Bit Operations/Bitwise Operator  logicop=AND  UseBitMask=on  BitMask=hex2dec('00000F00')  BitMaskRealWorld=Stored Integer
  SLOWNEWMSGDATAMASK_CNT_U32 : simulink/Logic and Bit Operations/Bitwise Operator  logicop=AND  UseBitMask=on  BitMask=hex2dec('80000000')  BitMaskRealWorld=Stored Integer
  Saturation : Saturate  UpperLimit=GearIdn1.EngMax  LowerLimit=GearIdn1.EngMin
      settings: AttributesFormatString=|
      | %<LowerLimit>
      | %<UpperLimit>
  SetNtcSts : Subsystem  RequirementInfo={'linktype_rmi_doors' '0000cf42 (/ESG Group/FDD Module Requirements/EA4 Specific/CM680A_HwTq2Meas)' '#CM680A_38' 'true' 'REQ: CM680A_38' '' } %GIDa_7c28da3a_b49c_4a2c_9776_430afb4b2413
  SlowSerlDataRead : Subsystem  RequirementInfo={'linktype_rmi_doors' '0000cf42 (/ESG Group/FDD Module Requirements/EA4 Specific/CM680A_HwTq2Meas)' '#CM680A_67' 'true' 'REQ: CM680A_67' '' } %GIDa_cfcf08de_2e21_4c55_8f79_af46abb48fdc
  TQDATAMASK_CNT_U32 : simulink/Logic and Bit Operations/Bitwise Operator  logicop=AND  UseBitMask=on  BitMask=hex2dec('00000FFF')  BitMaskRealWorld=Stored Integer
  Trq2ms : Scope  NumInputPorts=4
      settings: YMin=-10~0~1.9~0.95  YMax=10~275~2.1~1.05  SaveName=ScopeData3
  Unit Delay : UnitDelay  SampleTime=-1  StateName=HwTq2MeasPrevRollgCntr  StateMustResolveToSignalObject=on
      settings: AttributesFormatString=%<StateName>
  HwTq2 : Outport  RequirementInfo={} %GIDa_3b2abd0f_dff5_44f3_b788_adb2172836f5
  HwTq2Qlfr : Outport  RequirementInfo={'linktype_rmi_doors' '0000cf42 (/ESG Group/FDD Module Requirements/EA4 Specific/CM680A_HwTq2Meas)' '#CM680A_30' 'true' 'REQ: CM680A_30' '' } %GIDa_5eff5979_1038_44df_a727_ac7fcfb158b0  Port=2
  HwTq2RollgCntr : Outport  RequirementInfo={'linktype_rmi_doors' '0000cf42 (/ESG Group/FDD Module Requirements/EA4 Specific/CM680A_HwTq2Meas)' '#CM680A_31' 'true' 'REQ: CM680A_31' '' } %GIDa_de83414f_64c7_40b0_8047_6b8baba686d2  Port=3
  RegOutRSENT3CSC : Outport  Port=4
  GearIdn1Vld : Outport  RequirementInfo={} %GIDa_5a927bcd_e58c_45f1_b231_3df1879e401e  Port=5
  GearIdn1 : Outport  RequirementInfo={} %GIDa_ca1e138b_9ea0_4728_8c28_211cf335d6f4  Port=6
  wires:
  PrtclFltEvln/1(HwTqRaw) -> HwTqCalculation/1(RawHwTq)
  HwTqCalculation/1(HwTqData) -> PolarityEvaluation/1(HwTqData)
  PrtclFltEvln/2(TestOk) -> PolarityEvaluation/3(TestOk), RollCnt1/1(TestOk), Trq2ms/3, SetNtcSts/3(NtcSts), DebStepSelection/1(TestOk)  "TestOk"
  HwTq2Polarity/1 -> PolarityEvaluation/2(HwTq2Polarity)
  HwTq2PrtclFlt/1 -> SetNtcSts/1(NtcNr)  "NtcNr"
  PrtclFltEvln/3(ParamByte) -> SetNtcSts/2(NtcStInfo)  "ParamByte"
  HwTq2PrtclFlt1/1 -> GetNtcQlfr/1(NtcNr)
  DebStepSelection/1(DebStep) -> SetNtcSts/4(DebStep)
  FltInj_Sim1/1(Out1) -> Trq2ms/1, HwTq2/1  "HwTq2"
  RollCnt1/1(HwTq2RollgCntr) -> Unit Delay/1, Trq2ms/2, HwTq2RollgCntr/1  "HwTq2RollgCntr"
  Unit Delay/1 -> RollCnt1/2(HwTq2PrevRollgCntr)
  HwTq2MfgFlt/1 -> GetNtcQlfr1/1(NtcNr)
  GetNtcQlfr/1(NtcQlfr) -> If1/1
  GetNtcQlfr1/1(NtcQlfr) -> If1/2
  If Action Subsystem1/1(Qlfr) -> Merge1/1
  If Action Subsystem3/1(Qlfr) -> Merge1/2
  Merge1/1 -> Trq2ms/4, HwTq2Qlfr/1  "HwTq2Qlfr"
  If1/2 -> If Action Subsystem3/Action
  If1/1 -> If Action Subsystem1/Action
  FRSMASK_CNT_U32/1 -> PrtclFltEvln/1(HwTq2FRS)
  Data Type Conversion1/1 -> PrtclFltEvln/2(HwTq2CS)
  FCCNMASK_CNT_U32/1 -> PrtclFltEvln/3(HwTq2FCCN)
  TQDATAMASK_CNT_U32/1 -> PrtclFltEvln/4(HwTq2Data)
  FIU/1 -> FltInj_Sim1/2(Const)
  PolarityEvaluation/1(HwTq2) -> FltInj_Sim1/1(Signal)
  RegInpRSENT3FRS/1 -> If/1
  If/1 -> Read the Flag/Action
  If/2 -> Do nothing/Action
  RegInpRSENT3FND/1 -> Read the Flag/1(RegInpRSENT3FND)
  ClearFlag/1 -> RegOutRSENT3CSC/1
  CSMASK_CNT_U32/1 -> Data Type Conversion1/1
  RegInpRSENT3FRXD/1 -> SLOWNEWMSGDATAMASK_CNT_U32/1, TQDATAMASK_CNT_U32/1, FCCNMASK_CNT_U32/1
  RegInpRSENT3CS/1 -> SLOWCSMASK_ULS_U32/1, CSMASK_CNT_U32/1, FRSMASK_CNT_U32/1
  SlowSerlDataRead/1(GearIdn1Vld) -> GearIdn1Vld/1
  SlowSerlDataRead/2(GearIdn1) -> Saturation/1
  SLOWCSMASK_ULS_U32/1 -> SlowSerlDataRead/2(SlowSerlCS)
  SLOWNEWMSGDATAMASK_CNT_U32/1 -> SlowSerlDataRead/1(SlowSerlSND)
  RegInpRSENT3SRXD/1 -> SLOWMSGDATAMASK_CNT_U32/1, SLOWMSGIDMASK_CNT_U32/1
  SLOWMSGIDMASK_CNT_U32/1 -> RSHIFT8/1
  SLOWMSGDATAMASK_CNT_U32/1 -> Data Type Conversion3/1
  RSHIFT8/1 -> Data Type Conversion/1
  Data Type Conversion3/1 -> SlowSerlDataRead/4(SlowSerlMsgData)
  Data Type Conversion/1 -> SlowSerlDataRead/3(SlowSerlMsgID)
  Saturation/1 -> GearIdn1/1

== system CM680A_HwTq2Meas/HwTq2Meas/HwTq2MeasPer2 ==
  note: Information Only:
      | - Trim not performed Ntc
  function : TriggerPort  TriggerType=function-call
  CopyRight2 : Subsystem  Description=|  mask(Copyright Information){none=on}
      | Copyright info block.                                               
      |                                                                     
      | Place copyright information at the top of every subsystem in design.
      mask prompts: none "No parameters"
      mask help: Place copyright information at the top of every subsystem in design.
      mask Display:
      | NxtrConf = 'Nexteer Confidential';
      | 
      | sys = bdroot; %handle for the current model ("system")
      | first = get_param(sys,'Created');
      | first = first(end-3:end);  %year is last four digits
      | 
      | last = get_param(sys,'LastModifiedDate');
      | if isempty(last)
      |     last = datestr(now,'yyyy');
      | else
      |     last = last(end-3:end);
      | end
      | 
      | if strcmp(first,last)
      |     fprintf('%s -- Copyright %s Nexteer',NxtrConf,first)
      | else
      |     fprintf('%s -- %s%s- %s Nexteer',NxtrConf,char(169),first,last)
      | end
  Data Store Read1 : DataStoreRead  DataStoreName=HwTq2OffsTrimPrfmdSts
  Ground : Ground
  HwTq2MfgFlt : simulink/Sources/Enumerated Constant  OutDataTypeStr=Enum: NtcNr1  Value=NtcNr1.NTCNR_0X1E2  SampleTime=inf
  If : If  IfExpression=(u1 ~= 0)
  If Action Subsystem : Subsystem  RequirementInfo={'linktype_rmi_doors' '0000cf42 (/ESG Group/FDD Module Requirements/EA4 Specific/CM680A_HwTq2Meas)' '#CM680A_66' 'true' 'REQ: CM680A_66' '' } %GIDa_eda0e9fe_0ef4_4d37_918c_815346a1604f  TreatAsAtomicUnit=on
  If Action Subsystem1 : Subsystem  RequirementInfo={'linktype_rmi_doors' '0000cf42 (/ESG Group/FDD Module Requirements/EA4 Specific/CM680A_HwTq2Meas)' '#CM680A_64' 'true' 'REQ: CM680A_64' '' } %GIDa_f1a05e9a_fff8_4eab_8b85_2e72f495a740  TreatAsAtomicUnit=on
  Merge : Merge
  Merge1 : Merge
  Scope : Scope  NumInputPorts=2
      settings: YMin=-5~-5  YMax=5~5  SaveName=ScopeData3
  SetNtcSts : Subsystem  RequirementInfo={'linktype_rmi_doors' '0000cf42 (/ESG Group/FDD Module Requirements/EA4 Specific/CM680A_HwTq2Meas)' '#CM680A_60' 'true' 'REQ: CM680A_60' '' } %GIDa_03dde2fd_062f_4b23_859a_fc5579118954
  wires:
  Ground/1 -> SetNtcSts/4(DebStep)
  HwTq2MfgFlt/1 -> SetNtcSts/1(NtcNr)
  Data Store Read1/1 -> If/1
  If/1 -> If Action Subsystem/Action
  If/2 -> If Action Subsystem1/Action
  If Action Subsystem/1(ParamByte) -> Merge/1
  If Action Subsystem1/1(ParamByte) -> Merge/2
  If Action Subsystem/2(TestOk) -> Merge1/1
  If Action Subsystem1/2(TestOk) -> Merge1/2
  Merge/1 -> Scope/1, SetNtcSts/2(NtcStInfo)  "ParamByte"
  Merge1/1 -> Scope/2, SetNtcSts/3(NtcSts)  "TestOk"

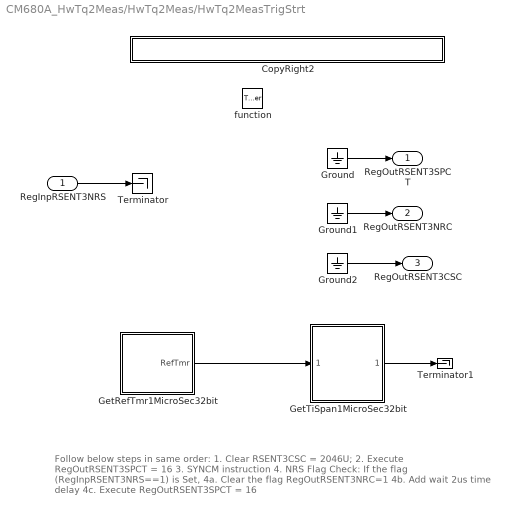
== system CM680A_HwTq2Meas/HwTq2Meas/HwTq2MeasTrigStrt ==
  note: Follow below steps in same order:
      |
      | 1. Clear RSENT3CSC = 2046U;
      | 2. Execute RegOutRSENT3SPCT = 16
      | 3. SYNCM instruction
      |
      | 4. NRS Flag Check: If the flag (RegInpRSENT3NRS==1) is Set,
      | 	4a. Clear the flag RegOutRSENT3NRC=1
      | 	4b. Add wait 2us time delay
      | 	4c. Execute RegOutRSENT3SPCT = 16
  RegInpRSENT3NRS : Inport
  function : TriggerPort  TriggerType=function-call
  CopyRight2 : Subsystem  Description=|  mask(Copyright Information){none=on}
      | Copyright info block.                                               
      |                                                                     
      | Place copyright information at the top of every subsystem in design.
      mask prompts: none "No parameters"
      mask help: Place copyright information at the top of every subsystem in design.
      mask Display:
      | NxtrConf = 'Nexteer Confidential';
      | 
      | sys = bdroot; %handle for the current model ("system")
      | first = get_param(sys,'Created');
      | first = first(end-3:end);  %year is last four digits
      | 
      | last = get_param(sys,'LastModifiedDate');
      | if isempty(last)
      |     last = datestr(now,'yyyy');
      | else
      |     last = last(end-3:end);
      | end
      | 
      | if strcmp(first,last)
      |     fprintf('%s -- Copyright %s Nexteer',NxtrConf,first)
      | else
      |     fprintf('%s -- %s%s- %s Nexteer',NxtrConf,char(169),first,last)
      | end
  GetRefTmr1MicroSec32bit : Subsystem
      settings: AttributesFormatString=Client Call : Start Time
  GetTiSpan1MicroSec32bit : Subsystem
  Ground : Ground
  Ground1 : Ground
  Ground2 : Ground
  Terminator : Terminator
  Terminator1 : Terminator
  RegOutRSENT3SPCT : Outport
  RegOutRSENT3NRC : Outport  Port=2
  RegOutRSENT3CSC : Outport  Port=3
  wires:
  Ground1/1 -> RegOutRSENT3NRC/1
  Ground/1 -> RegOutRSENT3SPCT/1
  Ground2/1 -> RegOutRSENT3CSC/1
  RegInpRSENT3NRS/1 -> Terminator/1
  GetTiSpan1MicroSec32bit/1(TiSpan) -> Terminator1/1
  GetRefTmr1MicroSec32bit/1(RefTmr) -> GetTiSpan1MicroSec32bit/1(RefTmr)

== system CM680A_HwTq2Meas/Simulated_Input/CopyRight2 ==
